simulink model "punto3modificado"  (R2017b)
settings: Solver=VariableStepAuto  StartTime=0.0  StopTime=.01  RelTol=1e-3
values from neighbouring files (symbols this model uses):
  kp = K    (= 60)    [Punto3.m]    (also in Punto4.m = 4)
  T0 = .1    (= 0.1)    [Punto1.m]    (also in Punto2.m = 2e-05; Punto4.m)
undefined symbols (not defined in the file or in its folder): dd, DiscIntNeverNeededParam, nd
libraries: simulink x1
settings Model: Creator=Agustin  LastModifiedBy=Agustin

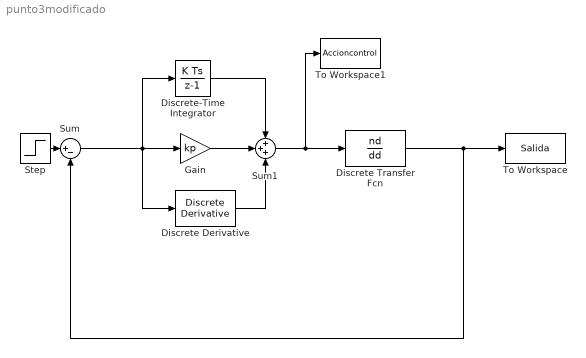
== system punto3modificado ==
  Discrete Transfer Fcn : DiscreteTransferFcn  Numerator=nd  Denominator=dd  SampleTime=T0
  Discrete Derivative : simulink/Discrete/Discrete Derivative  gainval=kd  ICPrevScaledInput=0.0  OutMin=[]  OutMax=[]  OutDataType=fixdt(1, 16)  OutScaling=2^-10  DoSatur=off
  Discrete-Time Integrator : DiscreteIntegrator  gainval=ki  InitialConditionSetting=State (most efficient)  SampleTime=T0  ICPrevOutput=DiscIntNeverNeededParam  ICPrevScaledInput=DiscIntNeverNeededParam
  Gain : Gain  Gain=kp
  Step : Step  Time=0  SampleTime=T0
  Sum : Sum  Inputs=|+-
  Sum1 : Sum  Inputs=+++
  To Workspace : ToWorkspace  VariableName=Salida  SaveFormat=Timeseries  SampleTime=-1
  To Workspace1 : ToWorkspace  VariableName=Accioncontrol  SaveFormat=Timeseries  SampleTime=-1
  wires:
  Discrete Transfer Fcn/1 -> To Workspace/1, Sum/2
  Step/1 -> Sum/1
  Sum/1 -> Discrete-Time Integrator/1, Discrete Derivative/1, Gain/1
  Discrete-Time Integrator/1 -> Sum1/1
  Gain/1 -> Sum1/2
  Discrete Derivative/1 -> Sum1/3
  Sum1/1 -> Discrete Transfer Fcn/1, To Workspace1/1
